simulink model "Roll_simulink_lqr"  (R2018b)
settings: Solver=VariableStepAuto  StartTime=0.0  StopTime=5  RelTol=1e-3
values from neighbouring files (symbols this model uses):
  Ar = [0,1;0,sin(beta)/Ixx*(N^2/R+c)*(-2*sin(beta)-Ixx/(Iw*sin(beta)))]    [Spacecraft.m]
  beta = 63.4*pi/180    (= 1.10653874576)    [Spacecraft.m]
  Br = [0;sin(beta)*N/(Ixx*R)]    [Spacecraft.m]
  Cr = [1,0;0,1]    [Spacecraft.m]
  Dr = [0;0]    [Spacecraft.m]
  int_resist = 6    [Spacecraft.m]
  Iw = max([Iw_roll Iw_pitch Iw_yaw])    [Spacecraft.m]    (also in maneuver.m = z2(end)*Is/(4*Omega_max*cos(beta)))
  Ixx = 6000    [Spacecraft.m]
  Kr = lqr(Ar,Br,Qr,Rr)    [Spacecraft.m]
  N = 60    [Spacecraft.m]
settings Model: Creator=Utilisateur  LastModifiedBy=Utilisateur

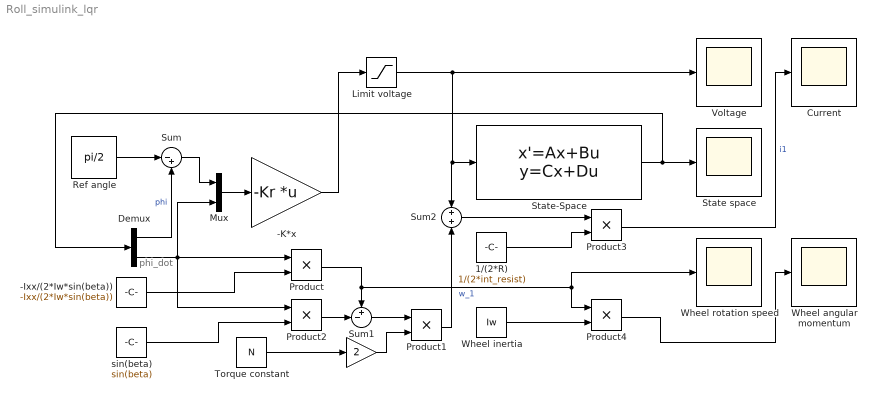
== system Roll_simulink_lqr ==
  note: phi_dot
  " " : Gain  Gain=2
  -Ixx/(2*Iw*sin(beta)) : Constant  Value=-Ixx/(2*Iw*sin(beta))
  "-K*x " : Gain  Gain=-Kr  Multiplication=Matrix(K*u) (u vector)
  1/(2*R) : Constant  Value=1/(2*int_resist)
  Current : Scope
  Demux : Demux  Outputs=2
  Limit voltage : Saturate  UpperLimit=387.5  LowerLimit=-387.5
  Mux : Mux  Inputs=2
  Product{,1..4} (5 alike) : Product
  Ref angle : Constant  Value=pi/2
  State space : Scope
  State-Space : StateSpace  A=Ar  B=Br  C=Cr  D=Dr  InitialCondition=[0;0]
  Sum : Sum  Inputs=|-+
  Sum1 : Sum  Inputs=+-|
  Sum2 : Sum  Inputs=+|+
  Torque constant : Constant  Value=N
  Voltage : Scope
  Wheel angular momentum : Scope
  Wheel inertia : Constant  Value=Iw
  Wheel rotation speed : Scope
  sin(beta) : Constant  Value=sin(beta)
  wires:
  Ref angle/1 -> Sum/1
  Sum/1 -> Mux/1
  Limit voltage/1 -> Sum2/1, State-Space/1, Voltage/1
  "-K*x "/1 -> Limit voltage/1
  Demux/1 -> Sum/2  "phi"
  Demux/2 -> Product/1, Mux/2, Product2/1
  Mux/1 -> "-K*x "/1
  State-Space/1 -> State space/1, Demux/1
  sin(beta)/1 -> Product2/2
  Product2/1 -> Sum1/2
  -Ixx/(2*Iw*sin(beta))/1 -> Product/2
  Product/1 -> Product4/1, Wheel rotation speed/1, Sum1/1  "w_1"
  Sum1/1 -> Product1/1
  Torque constant/1 -> " "/1
  " "/1 -> Product1/2
  Product1/1 -> Sum2/2
  Sum2/1 -> Product3/1
  1/(2*R)/1 -> Product3/2
  Product3/1 -> Current/1  "i1"
  Wheel inertia/1 -> Product4/2
  Product4/1 -> Wheel angular momentum/1
